simulink model "Plant_Model"  (R2021b)
settings: Solver=VariableStepAuto  StartTime=0.0  StopTime=10.0  RelTol=1e-3
values from neighbouring files (symbols this model uses):
  AirDensity_kgpm3 = 1.225    [vehicle_controller.mat]
  BatteryCapacity_Wh = 83    [vehicle_controller.mat]
  BatteryInitialEnergy = 58.1    [vehicle_controller.mat]
  BatteryMaxVoltage_V = 96    [vehicle_controller.mat]
  BatteryVoltageCoefficient_x = [0 0.1 0.2 0.3 0.4 0.5 0.6 0.7 0.8 0.9 1]    [vehicle_controller.mat]
  BatteryVoltageCoefficient_y = [0.833333333333 0.85 0.866666666667 0.883333333333 0.9 0.916666666667 0.933333333333 0.95 0.966666666667 0.983333333333 1]    [vehicle_controller.mat]
  BodyInitialSpeed_mps = 0    [vehicle_controller.mat]
  BodyMass_kg = 900    [vehicle_controller.mat]
  CombustionEngineMaxTorque_Nm = 100    [vehicle_controller.mat]
  DragArea_m2 = 4.5    [vehicle_controller.mat]
  DragCoeficient_1 = 0.4    [vehicle_controller.mat]
  FrictionCoefficient_Nsprad = 0.01    [vehicle_controller.mat]
  GearboxRatio_0_1 = 3    [vehicle_controller.mat]
  Ke = 0.1178    [vehicle_controller.mat]
  Kt = 0.668    [vehicle_controller.mat]
  L = looptransfer.Lo    [H_infinity_control_design.m]    (also in LoopShaping.m = G*K; Vehicle_Car_Controller.m = P * C)
  R = 0.141176    [vehicle_controller.mat]
  WheelDiameter_m = 0.5    [vehicle_controller.mat]
settings Model: Creator=beni  LastModifiedBy=beni

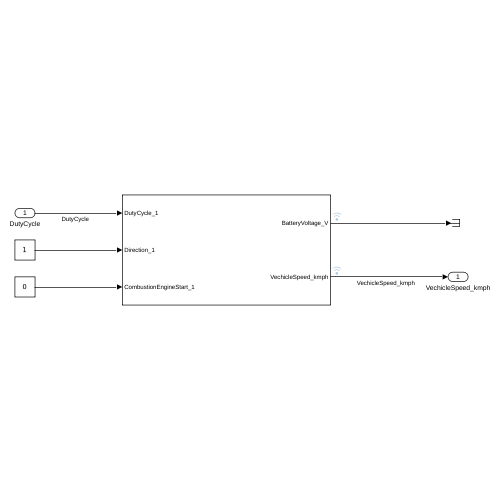
[thumbnail: Simulink's stored preview of the top-level diagram]
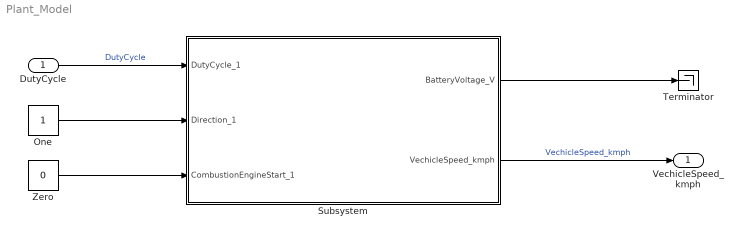
== system Plant_Model ==
  DutyCycle : Inport
  One : Constant  OutDataTypeStr=Inherit: Inherit via back propagation
  Subsystem : Subsystem
  Terminator : Terminator
  Zero : Constant  Value=0  OutDataTypeStr=Inherit: Inherit via back propagation
  VechicleSpeed_kmph : Outport
  wires:
  DutyCycle/1 -> Subsystem/1(DutyCycle_1)  "DutyCycle"
  One/1 -> Subsystem/2(Direction_1)
  Subsystem/1(BatteryVoltage_V) -> Terminator/1
  Subsystem/2(VechicleSpeed_kmph) -> VechicleSpeed_kmph/1  "VechicleSpeed_kmph"
  Zero/1 -> Subsystem/3(CombustionEngineStart_1)

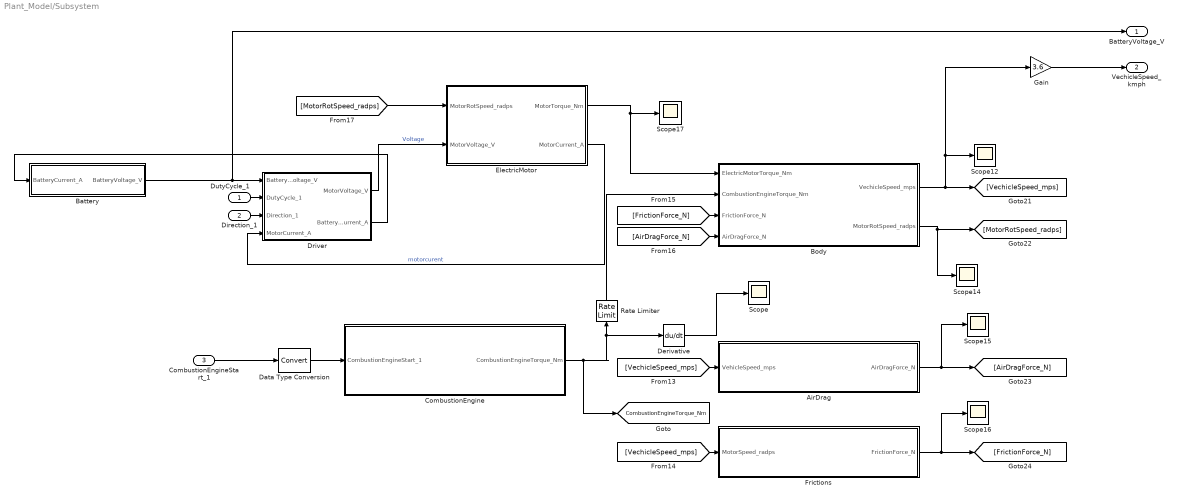
== system Plant_Model/Subsystem ==
  DutyCycle_1 : Inport
  Direction_1 : Inport  Port=2
  CombustionEngineStart_1 : Inport  Port=3
  AirDrag : Subsystem
  Battery : Subsystem
  Body : Subsystem
  CombustionEngine : Subsystem
  Data Type Conversion : DataTypeConversion
  Derivative : Derivative
  Driver : Subsystem
  ElectricMotor : Subsystem
  Frictions : Subsystem
  Gain : Gain  Gain=3.6
  Rate Limiter : RateLimiter  RisingSlewLimit=100  FallingSlewLimit=-100
  Scope{,12,14..17} (6 alike) : Scope
  BatteryVoltage_V : Outport
  VechicleSpeed_kmph : Outport  Port=2
  tag scope: CombustionEngineTorque_Nm=global
  wires:
  Direction_1/1 -> Driver/3(Direction_1)
  ElectricMotor/1(MotorTorque_Nm) -> Body/1(ElectricMotorTorque_Nm), Scope17/1
  [FrictionForce_N] -> Body/3(FrictionForce_N)
  Body/1(VechicleSpeed_mps) -> [VechicleSpeed_mps], Gain/1, Scope12/1
  Body/2(MotorRotSpeed_radps) -> Scope14/1, [MotorRotSpeed_radps]
  AirDrag/1(AirDragForce_N) -> [AirDragForce_N], Scope15/1
  Frictions/1(FrictionForce_N) -> Scope16/1, [FrictionForce_N]
  [VechicleSpeed_mps] -> AirDrag/1(VehicleSpeed_mps)
  Battery/1(BatteryVoltage_V) -> BatteryVoltage_V/1, Driver/1(BatteryVoltage_V)
  [AirDragForce_N] -> Body/4(AirDragForce_N)
  [MotorRotSpeed_radps] -> ElectricMotor/1(MotorRotSpeed_radps)
  [VechicleSpeed_mps] -> Frictions/1(MotorSpeed_radps)
  ElectricMotor/2(MotorCurrent_A) -> Driver/4(MotorCurrent_A)  "motorcurent"
  DutyCycle_1/1 -> Driver/2(DutyCycle_1)
  CombustionEngineStart_1/1 -> Data Type Conversion/1
  Gain/1 -> VechicleSpeed_kmph/1
  Data Type Conversion/1 -> CombustionEngine/1(CombustionEngineStart_1)
  Rate Limiter/1 -> Body/2(CombustionEngineTorque_Nm)
  Derivative/1 -> Scope/1
  Driver/2(BatteryCurrent_A) -> Battery/1(BatteryCurrent_A)
  CombustionEngine/1(CombustionEngineTorque_Nm) -> [CombustionEngineTorque_Nm], Derivative/1, Rate Limiter/1
  Driver/1(MotorVoltage_V) -> ElectricMotor/2(MotorVoltage_V)  "Voltage"

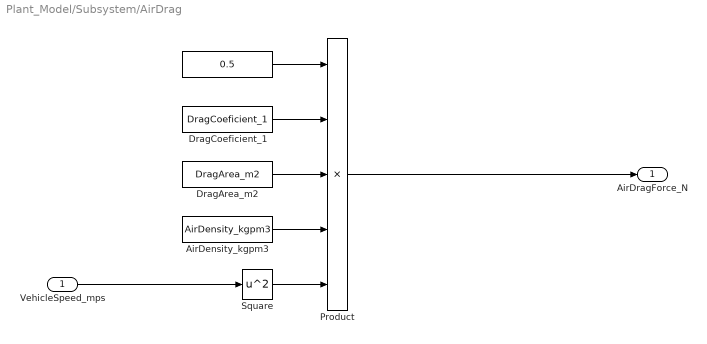
== system Plant_Model/Subsystem/AirDrag ==
  VehicleSpeed_mps : Inport
  " " : Constant  Value=0.5
  AirDensity_kgpm3 : Constant  Value=AirDensity_kgpm3
  DragArea_m2 : Constant  Value=DragArea_m2
  DragCoeficient_1 : Constant  Value=DragCoeficient_1
  Product : Product  Inputs=5
  Square : Math  Operator=square  SaturateOnIntegerOverflow=on
  AirDragForce_N : Outport
  wires:
  VehicleSpeed_mps/1 -> Square/1
  Square/1 -> Product/5
  DragArea_m2/1 -> Product/3
  AirDensity_kgpm3/1 -> Product/4
  DragCoeficient_1/1 -> Product/2
  " "/1 -> Product/1
  Product/1 -> AirDragForce_N/1

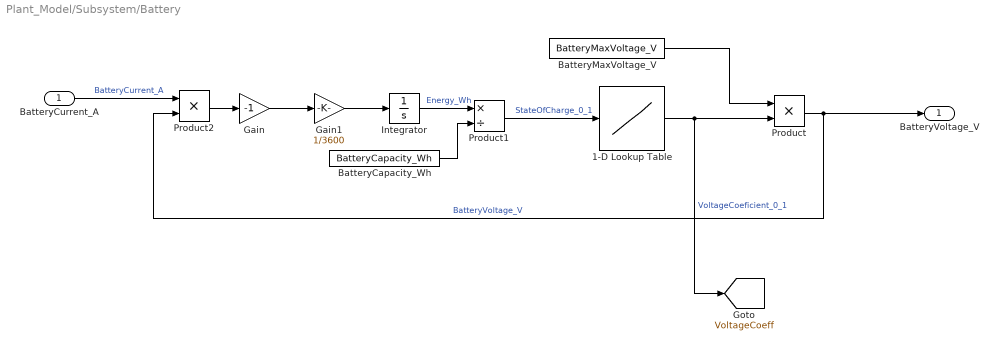
== system Plant_Model/Subsystem/Battery ==
  BatteryCurrent_A : Inport
  1-D Lookup Table : Lookup_n-D  NumberOfTableDimensions=1  BreakpointsForDimension1=BatteryVoltageCoefficient_x  Table=BatteryVoltageCoefficient_y  InternalRulePriority=Speed  RndMeth=Simplest  InputSameDT=on
  BatteryCapacity_Wh : Constant  Value=BatteryCapacity_Wh
  BatteryMaxVoltage_V : Constant  Value=BatteryMaxVoltage_V
  Gain : Gain  Gain=-1
  Gain1 : Gain  Gain=1/3600
  Integrator : Integrator  InitialCondition=BatteryInitialEnergy
  Product : Product
  Product1 : Product  Inputs=*/
  Product2 : Product
  BatteryVoltage_V : Outport
  tag scope: VoltageCoeff=global
  wires:
  BatteryCurrent_A/1 -> Product2/1  "BatteryCurrent_A"
  Product/1 -> Product2/2, BatteryVoltage_V/1  "BatteryVoltage_V"
  Integrator/1 -> Product1/1  "Energy_Wh"
  1-D Lookup Table/1 -> [VoltageCoeff], Product/2  "VoltageCoeficient_0_1"
  BatteryMaxVoltage_V/1 -> Product/1
  BatteryCapacity_Wh/1 -> Product1/2
  Product1/1 -> 1-D Lookup Table/1  "StateOfCharge_0_1"
  Product2/1 -> Gain/1
  Gain/1 -> Gain1/1
  Gain1/1 -> Integrator/1

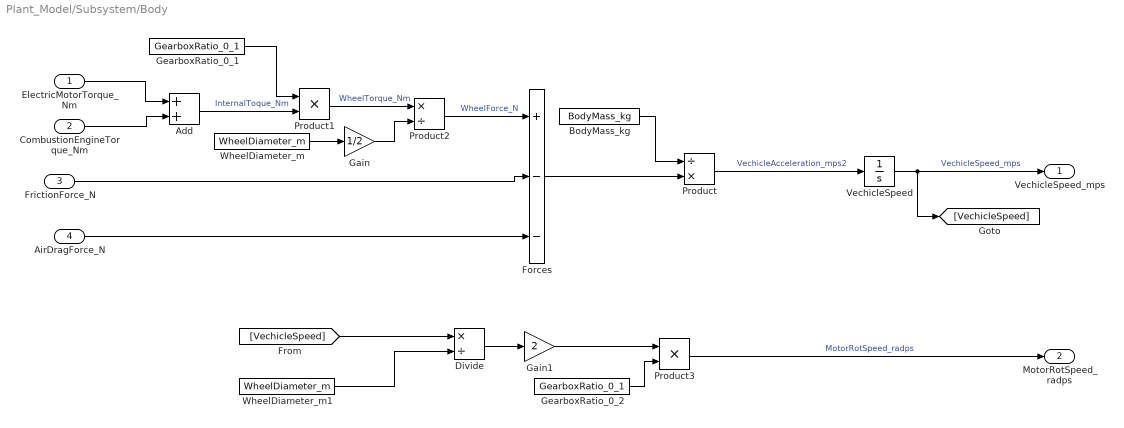
== system Plant_Model/Subsystem/Body ==
  ElectricMotorTorque_Nm : Inport
  CombustionEngineTorque_Nm : Inport  Port=2
  FrictionForce_N : Inport  Port=3
  AirDragForce_N : Inport  Port=4
  Add : Sum
  BodyMass_kg : Constant  Value=BodyMass_kg
  Divide : Product  Inputs=*/
  Forces : Sum  Inputs=+--
  Gain : Gain  Gain=1/2
  Gain1 : Gain  Gain=2
  GearboxRatio_0_1 : Constant  Value=GearboxRatio_0_1
  GearboxRatio_0_2 : Constant  Value=GearboxRatio_0_1
  Product : Product  Inputs=/*
  Product1 : Product
  Product2 : Product  Inputs=*/
  Product3 : Product  Inputs=**
  VechicleSpeed : Integrator  InitialCondition=BodyInitialSpeed_mps
  WheelDiameter_m : Constant  Value=WheelDiameter_m
  WheelDiameter_m1 : Constant  Value=WheelDiameter_m
  VechicleSpeed_mps : Outport
  MotorRotSpeed_radps : Outport  Port=2
  wires:
  VechicleSpeed/1 -> [VechicleSpeed], VechicleSpeed_mps/1  "VechicleSpeed_mps"
  Product/1 -> VechicleSpeed/1  "VechicleAcceleration_mps2"
  BodyMass_kg/1 -> Product/1
  Forces/1 -> Product/2
  AirDragForce_N/1 -> Forces/3
  FrictionForce_N/1 -> Forces/2
  ElectricMotorTorque_Nm/1 -> Add/1
  CombustionEngineTorque_Nm/1 -> Add/2
  Add/1 -> Product1/2  "InternalToque_Nm"
  GearboxRatio_0_1/1 -> Product1/1
  Product1/1 -> Product2/1  "WheelTorque_Nm"
  WheelDiameter_m/1 -> Gain/1
  Product2/1 -> Forces/1  "WheelForce_N"
  Gain/1 -> Product2/2
  [VechicleSpeed] -> Divide/1
  WheelDiameter_m1/1 -> Divide/2
  Divide/1 -> Gain1/1
  Gain1/1 -> Product3/1
  GearboxRatio_0_2/1 -> Product3/2
  Product3/1 -> MotorRotSpeed_radps/1  "MotorRotSpeed_radps"

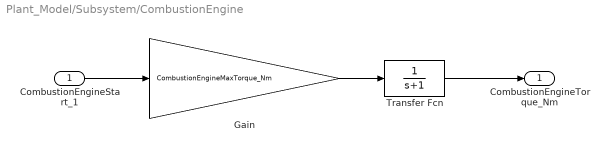
== system Plant_Model/Subsystem/CombustionEngine ==
  CombustionEngineStart_1 : Inport
  Gain : Gain  Gain=CombustionEngineMaxTorque_Nm
  Transfer Fcn : TransferFcn  Denominator=[1 1]
  CombustionEngineTorque_Nm : Outport
  wires:
  Transfer Fcn/1 -> CombustionEngineTorque_Nm/1
  CombustionEngineStart_1/1 -> Gain/1
  Gain/1 -> Transfer Fcn/1

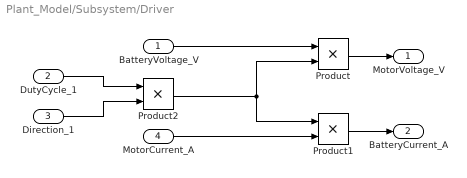
== system Plant_Model/Subsystem/Driver ==
  BatteryVoltage_V : Inport
  DutyCycle_1 : Inport  Port=2
  Direction_1 : Inport  Port=3
  MotorCurrent_A : Inport  Port=4
  Product : Product
  Product1 : Product
  Product2 : Product
  MotorVoltage_V : Outport
  BatteryCurrent_A : Outport  Port=2
  wires:
  BatteryVoltage_V/1 -> Product/1
  Product/1 -> MotorVoltage_V/1
  Product2/1 -> Product1/1, Product/2
  MotorCurrent_A/1 -> Product1/2
  Product1/1 -> BatteryCurrent_A/1
  DutyCycle_1/1 -> Product2/1
  Direction_1/1 -> Product2/2

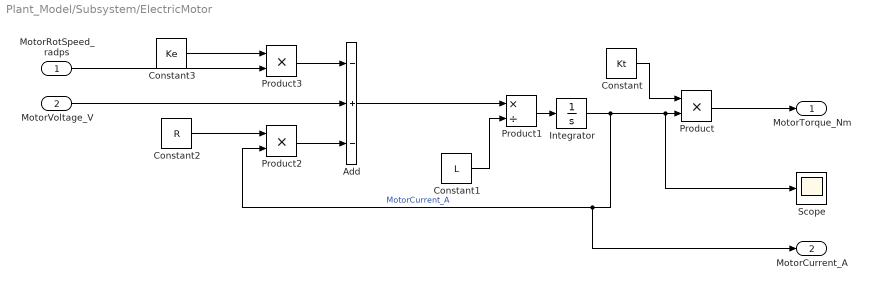
== system Plant_Model/Subsystem/ElectricMotor ==
  MotorRotSpeed_radps : Inport
  MotorVoltage_V : Inport  Port=2
  Add : Sum  Inputs=-+-
  Constant : Constant  Value=Kt
  Constant1 : Constant  Value=L
  Constant2 : Constant  Value=R
  Constant3 : Constant  Value=Ke
  Integrator : Integrator
  Product : Product
  Product1 : Product  Inputs=*/
  Product2 : Product
  Product3 : Product
  Scope : Scope
  MotorTorque_Nm : Outport
  MotorCurrent_A : Outport  Port=2
  wires:
  Product/1 -> MotorTorque_Nm/1
  Integrator/1 -> MotorCurrent_A/1, Product2/2, Scope/1, Product/2  "MotorCurrent_A"
  Constant/1 -> Product/1
  Product1/1 -> Integrator/1
  Constant1/1 -> Product1/2
  Add/1 -> Product1/1
  Product2/1 -> Add/3
  Constant2/1 -> Product2/1
  MotorVoltage_V/1 -> Add/2
  Constant3/1 -> Product3/1
  Product3/1 -> Add/1
  MotorRotSpeed_radps/1 -> Product3/2

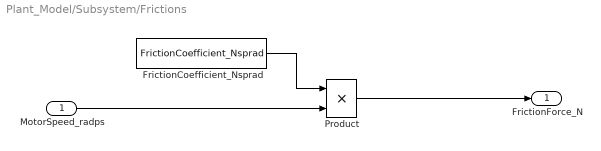
== system Plant_Model/Subsystem/Frictions ==
  MotorSpeed_radps : Inport
  FrictionCoefficient_Nsprad : Constant  Value=FrictionCoefficient_Nsprad
  Product : Product
  FrictionForce_N : Outport
  wires:
  Product/1 -> FrictionForce_N/1
  MotorSpeed_radps/1 -> Product/2
  FrictionCoefficient_Nsprad/1 -> Product/1
